simulink library "read"  (R2024a)
settings: Solver=VariableStepAuto  StartTime=0.0  StopTime=10.0  RelTol=1e-3
settings Model: Creator=eikel  LastModifiedBy=eikel

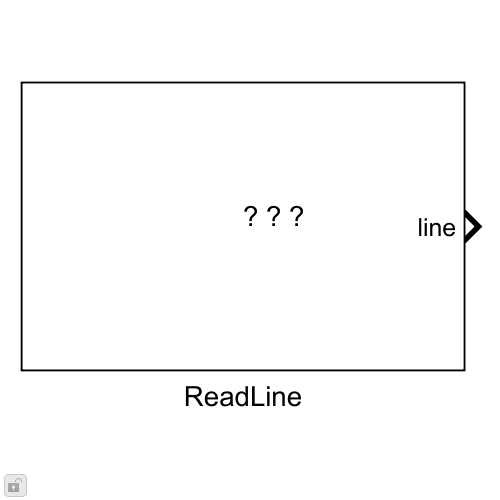
[thumbnail: Simulink's stored preview of the top-level diagram]
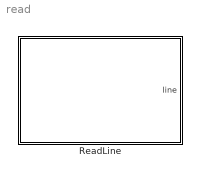
== system read ==
  ReadLine : Subsystem
      mask Display: image('lineDetector.jpg');

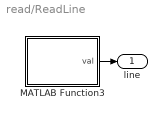
== system read/ReadLine ==
  MATLAB Function3 : MATLAB Function  TreatAsAtomicUnit=on
  line : Outport
  wires:
  MATLAB Function3/1(val) -> line/1

== matlab function read/ReadLine/MATLAB Function3 ==
  data: val output
function val = read_line()
    coder.extrinsic('get_line');  % merk: dette peikar på .m-fila di
    val =0;                         % initier output
    val = get_line();            % kall den eksterne funksjonen
end
